simulink model "power_hvdc12pulse"  (Simulink 6.0)
settings: Solver=FixedStepDiscrete  SolverMode=SingleTasking  StartTime=0.0  StopTime=2  FixedStep=Ts  RelTol=1e-3  AbsTol=1e-2
InitFcn:
  | Ts=50e-6;
undefined symbols (not defined in the file or in its folder): CLARK, Current, D1, Delta, DiscIntNeverNeededParam, Gamma, Inverter, lag, lib_mesures, Voltage, Yg
libraries: powerlib x39, powerlib_extras x30, simulink x3
(part 2 of 3)

== system power_hvdc12pulse/Inverter Control and Protection/Inverter Protections ==
  Uabc (pu) : Inport  Port=1  LatchInput=off
  1st-Order T=3.3 ms : powerlib_extras/Discrete  Control Blocks/Discrete 1st-Order Discrete Filter  FilterType=Lowpass  Tc=0.0033  Ts=Ts  Initialize=off  Vac_Init=[0.8 -25 60]  Vdc_Init=-0.4  PlotResponse=off  param1=[1 500 0.1]
  Commutation Failure Prevention Control (CFPREV) : Subsystem  mask(Commutation Failure Prevention Control){STATE=on, T_ss=0.64, ab_level=0.1, ab_gain=25, z_level=0.1, z_gain=25, fn=60, Filter=[2.0, 1.0], Ts=Ts}
      mask prompts: STATE "ON State"; T_ss "Simulation Steady_State Time (s):"; ab_level "ab level (pu):"; ab_gain "ab gain (deg/pu):"; z_level "z level (pu):"; z_gain "z gain (deg/pu):"; fn "Base frequency (Hz):"; Filter "Filter Time const. and Iinitial condition [T(s), Ic (pu)]:"; Ts "Sample Time (s):"
      mask help:
      | The protective function, used in the inverter, mitigates commutation failures due to AC voltage dips. After a fault detection (three-phase or one-phase) an angle value (AMIN_CFPREV) is sent to the converter control in order to be deducted from the maximum delay angle limit (alpha_max). Practicaly, the commutation margin is consequently enlarged reducing therfore the risk of commutation failures.
      |
      |      The CLARK transformation is used for three-phase fault  detection and the zero-sequence voltage evaluation. The detection is based  on instantaneous values, which ensure fast reaction of the control system when AC faults occurs.
      |
      |      Press Help to get the reference with the  detailed description of the function and  parameters.
      |
      | Note: To accelerate the function initialisation, the first parameter (Simulation Steady_State Time) is used. It corresponds to the time when the input voltages reache  the steady-state value.
      mask init:
      | T_periode = 0.6/fn;    % More then half the period
      | filt_tc = Filter(1);
      | filt_ic = Filter(2);
      | 
      | if (STATE)
      | 	str = 'ON';
      | else
      | 	str = 'OFF';
      | end
      mask Help:
      | Ref. "A Novel Method to Mitigate Commutation Failures in HVDC Systems,"
      | Lidong Zhang, Lars Dofnas ABB Utilities Power System Technology,
      | Proceedings PowerCon 2002, Volume: 1 , 13-17 Oct. 2002,  Page(s): 51-56 vol.1.
      mask Display: disp(['\n\n\n State:[',str,']'])
  Informations : Subsystem
      mask Display: disp('?')
  Low AC Voltage Detection (LACVD) : Subsystem  TreatAsAtomicUnit=on  mask(Low AC voltage detection){STATE=on, Ref_1=0.75, dt=fix(0.001/Ts)*Ts}
      mask prompts: STATE "ON State"; Ref_1 "Detection level (pu):"; dt "Sample time (s):"
      mask help:
      | This bloc detects a low AC voltage condition on the commutation busbar and is used in the DC protection scheme. Its purpose is to descriminate between a drop in the AC voltage caused by a fault on the DC line or by a fault on the AC side.
      |
      |      An AC fault detection (Low_ac_voltage output signal) will occur when the AC voltage input (recified three-phase AC voltage) drops below a certain reference value (Detection
      | level).
      |
      |      In order to minimize the simulation time, an enabled susbystem having a sample time of 1 (ms) has been used in accordance with an acceptable precision.
      mask init:
      | if (STATE)
      | 	str = 'ON';
      | else
      | 	str = 'OFF';
      | end
      mask Display: disp(['\n\n\n\nState:[',str,']'])
  T = 1 ms : DiscretePulseGenerator  Period=fix(0.001/Ts)  SampleTime=Ts
  Udio_6p : Subsystem
  Low_AC_Voltage : Outport
  AMIN_CFPREV : Outport  Port=2
  wires:
  T = 1 ms/1 -> Low AC Voltage Detection (LACVD)/Enable
  1st-Order T=3.3 ms/1 -> Low AC Voltage Detection (LACVD)/1(Uac (pu))
  Udio_6p/1(Udio_6p) -> 1st-Order T=3.3 ms/1
  Uabc (pu)/1 -> Commutation Failure Prevention Control (CFPREV)/1(Uabc (pu)), Udio_6p/1(Uabc (pu))
  Low AC Voltage Detection (LACVD)/1(Low_AC_Voltage) -> Low_AC_Voltage/1
  Commutation Failure Prevention Control (CFPREV)/1(AMIN_CFPREV (deg)) -> AMIN_CFPREV/1

== system power_hvdc12pulse/Master Control/Informations ==
  note: For testing purpose,  a step can be activated and added to the reference current at both
      | converters.
  note: Master Control
  note: INTRODUCTION
  note: The rectifier and inverter current reference are generated in the master control. The reference
      | should be equal in both converters to avoid the loss of the margin. The converter starting and stopping is
      | initiated and the current reference can be ramped up or down.  A current step can be added to the
      | current reference for testing purpose.
  note: DESCRIPTION
  note: At start-up, both converters are deblocked and ramped up to the minimum current allowed in steady-state
      | with an adjustable rate  and application time in the "Start/Stop & Ramping Unit" subsystem. After the
      | system stabilisation the current is ramped up to its final value  with an adjustable rate and execution time.
      | Before stopping the converters the current is ramped down to the minimum reference.

== system power_hvdc12pulse/Master Control/Start/Stop ==
  note: Start/Stop sequence
  note: Start/Stop & Ramping
  note: Ramping
  Discrete Bistable : powerlib_extras/Discrete  Control Blocks/Discrete Bistable  Priority=0  ic=0  Ts=50e-6
  Discrete Edge Detector1 : powerlib_extras/Discrete  Control Blocks/Discrete Edge Detector  model=Rising  ic=0  Ts=Ts
  Discrete Edge Detector2 : powerlib_extras/Discrete  Control Blocks/Discrete Edge Detector  model=Rising  ic=0  Ts=Ts
  Logical Operator3 : Logic  AllPortsSameDT=off
  Minimum ref : Constant  Value=Min_ref
  Relational Operator1 : RelationalOperator  Operator=<=
  S1 : Subsystem  mask(RAMPING UNIT){Min_ref=Min_ref, SS_ramp=SS_ramp, F_up=F_up, up_slope=up_slope, T_up=T_up, F_down=F_down, down_slope=down_slope, T_down=T_down}
      mask prompts: Min_ref "Minimum Value (pu):"; SS_ramp "Start-Stop ramp (pu/s):"; F_up "Final Up Value (pu):"; up_slope "Up Slope (pu/s):"; T_up "Ramping Up Time (s):"; F_down "Final Down Value (pu):"; down_slope "Down Slope (pu/s):"; T_down "Ramping Down Time (s):"
      mask init:
      | T_up_final      =  T_up + (F_up - Min_ref)/up_slope;
      | T_down_final =   T_down + (F_down-F_up)/down_slope;
      | T_ramp  = [0, T_up, T_up_final,  T_down,  T_down_final, 9999]';
      | U_ramp = [0, 0, F_up-Min_ref,  F_up-Min_ref,  F_down- Min_ref,  F_down - Min_ref]';
      mask Display: disp('Ramping\n Unit')
  Start : Step  Time=T_start  SampleTime=0
  Stop : Step  Time=T_stop  SampleTime=0
  Unit Delay : UnitDelay  Orientation=left  SampleTime=Ts
  Id_ref_ramp : Outport
  "Stop " : Outport  Port=2
  wires:
  Discrete Edge Detector2/1 -> Discrete Bistable/2
  S1/1(Out1) -> Unit Delay/1, Id_ref_ramp/1
  Discrete Bistable/2 -> "Stop "/1
  Minimum ref/1 -> Relational Operator1/2
  Unit Delay/1 -> Relational Operator1/1
  Start/1 -> Discrete Edge Detector1/1
  Discrete Bistable/1 -> S1/1(Start)  "Start"
  Logical Operator3/1 -> Discrete Edge Detector2/1
  Relational Operator1/1 -> Logical Operator3/1
  Stop/1 -> Logical Operator3/2
  Discrete Edge Detector1/1 -> Discrete Bistable/1

== system power_hvdc12pulse/Rectifier/Rectifier ==
  Py : Inport  Port=1  LatchInput=off
  Pd : Inport  Port=2  LatchInput=off
  Bridge D : powerlib/Power Electronics/Universal Bridge  Arms=3  SnubberResistance=2000  SnubberCapacitance=0.1e-6  Device=Thyristors  Ron=1e-3  Lon=0  ForwardVoltages="[  0.8  0.8  ]"  ForwardVoltage=0  GTOparameters=[ 10e-6 , 20e-6 ]  IGBTparameters=[ 1e-6 , 2e-6 ]  Measurements=None
  Bridge Y : powerlib/Power Electronics/Universal Bridge  Arms=3  SnubberResistance=2000  SnubberCapacitance=0.1e-6  Device=Thyristors  Ron=1e-3  Lon=0  ForwardVoltages="[  0.8  0.8  ]"  ForwardVoltage=0  GTOparameters=[ 10e-6 , 20e-6 ]  IGBTparameters=[ 1e-6 , 2e-6 ]  Measurements=All voltages and currents
  Ay : PMIOPort  Port=1  Side=Left
  By : PMIOPort  Port=2  Side=Left
  Cy : PMIOPort  Port=3  Side=Left
  Ad : PMIOPort  Port=4  Side=Left
  Bd : PMIOPort  Port=5  Side=Left
  Cd : PMIOPort  Port=6  Side=Left
  pos : PMIOPort  Orientation=left  Port=7  Side=Right
  neg : PMIOPort  Orientation=left  Port=8  Side=Right
  wires:
  Pd/1 -> Bridge D/1
  Py/1 -> Bridge Y/1
  connections:
  Bridge D/RConn2 -- neg/RConn1
  Cd/RConn1 -- Bridge D/LConn3
  Bd/RConn1 -- Bridge D/LConn2
  Ad/RConn1 -- Bridge D/LConn1
  Cy/RConn1 -- Bridge Y/LConn3
  By/RConn1 -- Bridge Y/LConn2
  Bridge Y/RConn1 -- pos/RConn1
  Ay/RConn1 -- Bridge Y/LConn1
  Bridge D/RConn1 -- Bridge Y/RConn2

== system power_hvdc12pulse/Rectifier Control and Protection/12-pulse Firing Control1 ==
  alpha_ord (deg) : Inport  Port=1  LatchInput=off
  Vabc (pu) : Inport  Port=2  LatchInput=off
  Block : Inport  Port=3  LatchInput=off
  Discrete Synchronized 12-Pulse Generator : Subsystem  AncestorBlock=|  mask(Discrete synchronized 12-pulse generator){pwidth=Pw, Double_Pulse=off, Ts=dt}
      | powerlib_extras/Discrete 
      | Control Blocks/Discrete Synchronized
      | 12-Pulse Generator
      mask prompts: pwidth "Pulse width (degrees) :"; Double_Pulse "Double pulsing"; Ts "Sample time:"
      mask help:
      | Use his block  to fire the 12 thyristors of a 12-pulse converter.
      | Outputs 1 and 2 are two vectors of 6 pulses (0-1) to be sent to the two 6-pulse half bridges connected respectively to the Wye(Y) and Delta (D) connected windings of the YYD converter transformer. Pulses are individually synchronized on the 6 commutation voltages and generated alpha degrees after the increasing zero-crossings of the commutation voltages. The D pulses are lagging the Y pulses by  60 degrees.
      |
      | Input 1 is  the alpha firing signal (degrees).
      | Inputs 2, 3 and 4 are the three phase-ground synchronization voltages  measured at the  primary side of the converter transformer.
      | Input 5: Frequency of the synchronization voltages (use a constant or the Freq PLL output)
      | Input 6 allows  blocking of the pulses when the applied signal is non zero.
      |
      | When the 'Douple pulsing' option is checked, two pulses are sent to each thyristor: a 1st pulse when the aplha angle is reached, then a 2nd pulse 60 degrees later, when the next thyristor is fired.
      mask Display: plot(0,0,100,100,[80 62 62 47 47 30],[40 40 60 60 40 40]-5)
  PLL : Subsystem
  PulsesY : Outport
  PulsesD : Outport  Port=2
  Freq : Outport  Port=3
  wires:
  Discrete Synchronized 12-Pulse Generator/1(PY) -> PulsesY/1
  Discrete Synchronized 12-Pulse Generator/2(PD) -> PulsesD/1
  Vabc (pu)/1 -> PLL/1(Vabc(pu))
  PLL/1(Va) -> Discrete Synchronized 12-Pulse Generator/2(A)
  PLL/2(Vb) -> Discrete Synchronized 12-Pulse Generator/3(B)
  PLL/3(Vc) -> Discrete Synchronized 12-Pulse Generator/4(C)
  PLL/4(Freq) -> Discrete Synchronized 12-Pulse Generator/5(Freq), Freq/1
  alpha_ord (deg)/1 -> Discrete Synchronized 12-Pulse Generator/1(alpha_deg)
  Block/1 -> Discrete Synchronized 12-Pulse Generator/6(Block)

== system power_hvdc12pulse/Rectifier Control and Protection/Rectifier Protections ==
  note: DC Protections (in Rectifier)
  Uabc (pu) : Inport  Port=1  LatchInput=off
  VdL (pu) : Inport  Port=2  LatchInput=off
  Deblocked : Inport  Port=3  LatchInput=off
  Low_ac_volt_oth : Inport  Port=4  LatchInput=off
  1st-Order T=3.3 ms : powerlib_extras/Discrete  Control Blocks/Discrete 1st-Order Discrete Filter  FilterType=Lowpass  Tc=0.0033  Ts=Ts  Initialize=off  Vac_Init=[0.8 -25 60]  Vdc_Init=-0.4  PlotResponse=off  param1=[1 500 0.1]
  DC Fault Protection (DCPROT) : Subsystem  mask(DC fault protection (in Rectifier)){STATE=on, Ref1=0.5, T1=0.070, T2=0.05, polarity=Positive, dt=fix(0.002/Ts)*Ts}
      mask prompts: STATE "ON State"; Ref1 "Detection level (pu):"; T1 "Detection delay (s):"; T2 "Forced alpha duration (s):"; polarity "Voltage polarity:"; dt "Sample time (s):"
      mask help:
      | The protection is active in the rectifier. It will detect a fault on the DC side and will force the delay angle into the inverter region in order to extinguish the fault current.
      |      The fault detection on the DC line is based on the drop in the line to ground voltage.
      |      The normal voltage polarity (+ or -) of the line is a parameter as well as the reference level (Detection level) of the fault detection.
      |      A delay time (Detection delay) is used in the detection to descriminate between a line fault and other disturbances resulting in a low DC voltage.
      |      A delay time (200 ms) is allowed, after the DC system start-up, before activating the detection logic to make sure that the normal operating DC voltage is established.
      |      Also, an external signal (Lock) generated by another protective function (e.g. Low AC voltage detection) will lock the detection for a minimum amount of time (set by an Off Delay bloc) in order to descriminate between any fault causing a low DC voltage.
      |      A detection will triger a Forced alpha during an ajustable interval (Forced alpha duration) sufficient to allow for deionization of the fault path prior to re-application of voltage.
      |
      |      In order to minimize the simulation time, an enabled susbystem having a sample time of  2 (ms) has been used in accordance with an acceptable precision.
      mask init:
      | if (polarity == 1)
      | 	sign = 1;
      | else
      | 	sign = -1;
      | end
      | 
      | if (STATE)
      | 	str = 'ON';
      | else
      | 	str = 'OFF';
      | end
      mask StyleString: checkbox,edit,edit,edit,popup(Positive|Negative),edit
      mask Display: disp(['\n\n\n\nState:[',str,']'])
  Informations : Subsystem
      mask Display: disp('?')
  Logical Operator6 : Logic  Operator=OR
  Low AC Voltage Detection (LACVD) : Subsystem  TreatAsAtomicUnit=on  mask(Low AC voltage detection){STATE=on, Ref_1=0.70, dt=fix(0.001/Ts)*Ts}
      mask prompts: STATE "ON State"; Ref_1 "Detection level (pu):"; dt "Sample time (s):"
      mask help:
      | This bloc detects a low AC voltage condition on the commutation busbar and is used in the DC protection scheme. Its purpose is to descriminate between a drop in the AC voltage caused by a fault on the DC line or by a fault on the AC side.
      |
      |      An AC fault detection (Low_ac_voltage output signal) will occur when the AC voltage input (recified three-phase AC voltage) drops below a certain reference value (Detection level).
      |
      |      In order to minimize the simulation time, an enabled susbystem having a sample time of 1 (ms) has been used in accordance with an acceptable precision.
      mask init:
      | if (STATE)
      | 	str = 'ON';
      | else
      | 	str = 'OFF';
      | end
      mask Display: disp(['\n\n\n\nState:[',str,']'])
  T = 1 ms : DiscretePulseGenerator  Period=fix(0.001/Ts)  SampleTime=Ts
  T = 2 ms : DiscretePulseGenerator  Period=fix(0.002/Ts)  SampleTime=Ts
  Udio_6p : Subsystem
  Forced_alpha : Outport
  Low_ac_voltage : Outport  Port=2
  wires:
  T = 1 ms/1 -> Low AC Voltage Detection (LACVD)/Enable
  1st-Order T=3.3 ms/1 -> Low AC Voltage Detection (LACVD)/1(Uac (pu))
  Udio_6p/1(Udio_6p) -> 1st-Order T=3.3 ms/1
  Uabc (pu)/1 -> Udio_6p/1(Uabc (pu))
  Low AC Voltage Detection (LACVD)/1(Low_AC_Voltage) -> Logical Operator6/1, Low_ac_voltage/1
  T = 2 ms/1 -> DC Fault Protection (DCPROT)/Enable
  DC Fault Protection (DCPROT)/1(Forced_alpha) -> Forced_alpha/1
  Low_ac_volt_oth/1 -> Logical Operator6/2
  Logical Operator6/1 -> DC Fault Protection (DCPROT)/3(Lock)
  VdL (pu)/1 -> DC Fault Protection (DCPROT)/1(VdL (pu))
  Deblocked/1 -> DC Fault Protection (DCPROT)/2(Deblocked)

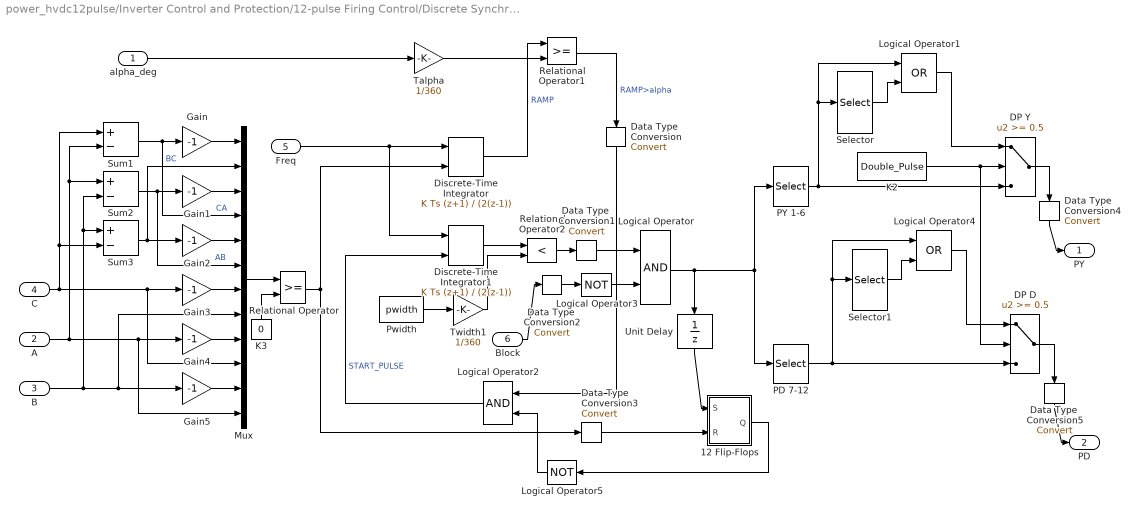
== system power_hvdc12pulse/Inverter Control and Protection/12-pulse Firing Control/Discrete Synchronized 12-Pulse Generator ==
  alpha_deg : Inport  Port=1  LatchInput=off
  A : Inport  Port=2  LatchInput=off
  B : Inport  Port=3  LatchInput=off
  C : Inport  Port=4  LatchInput=off
  Freq : Inport  Port=5  LatchInput=off
  Block : Inport  Port=6  LatchInput=off
  12 Flip-Flops : Subsystem
  DP D : Switch  Threshold=0.5  InputSameDT=on
  DP Y : Switch  Threshold=0.5  InputSameDT=on
  Data Type  Conversion : DataTypeConversion  Orientation=down  OutDataTypeMode=boolean  SaturateOnIntegerOverflow=on  RndMeth=Zero
  Data Type  Conversion1 : DataTypeConversion  OutDataTypeMode=boolean  SaturateOnIntegerOverflow=on  RndMeth=Zero
  Data Type  Conversion2 : DataTypeConversion  OutDataTypeMode=boolean  SaturateOnIntegerOverflow=on  RndMeth=Zero
  Data Type  Conversion3 : DataTypeConversion  OutDataTypeMode=boolean  SaturateOnIntegerOverflow=on  RndMeth=Zero
  Data Type  Conversion4 : DataTypeConversion  Orientation=down  OutDataTypeMode=double  SaturateOnIntegerOverflow=on  RndMeth=Zero
  Data Type  Conversion5 : DataTypeConversion  Orientation=down  OutDataTypeMode=double  SaturateOnIntegerOverflow=on  RndMeth=Zero
  Discrete-Time Integrator : DiscreteIntegrator  IntegratorMethod=Integration: Trapezoidal  ExternalReset=rising  SampleTime=Ts  ICPrevOutput=DiscIntNeverNeededParam  ICPrevScaledInput=DiscIntNeverNeededParam
  Discrete-Time Integrator1 : DiscreteIntegrator  IntegratorMethod=Integration: Trapezoidal  ExternalReset=rising  SampleTime=Ts  ICPrevOutput=DiscIntNeverNeededParam  ICPrevScaledInput=DiscIntNeverNeededParam
  Gain{,1..5} (6 alike) : Gain  Gain=-1  SaturateOnIntegerOverflow=on
  K2 : Constant  Value=Double_Pulse
  K3 : Constant  Orientation=up  Value=0
  Logical Operator : Logic
  Logical Operator1 : Logic  Operator=OR
  Logical Operator2 : Logic  Orientation=left
  Logical Operator3 : Logic  Operator=NOT  Inputs=1
  Logical Operator4 : Logic  Operator=OR
  Logical Operator5 : Logic  Orientation=left  Operator=NOT  Inputs=1
  Mux : Mux  Inputs=12
  PD 7-12 : Selector  Elements=7:12  InputPortWidth=12
  PY 1-6 : Selector  Elements=1:6  InputPortWidth=12
  Pwidth : Constant  Value=pwidth
  Relational Operator : RelationalOperator  InputSameDT=on
  Relational Operator1 : RelationalOperator  InputSameDT=on
  Relational Operator2 : RelationalOperator  Operator=<  InputSameDT=on
  Selector : Selector  Elements=[2 3 4 5 6 1 ]  InputPortWidth=6
  Selector1 : Selector  Elements=[2 3 4 5 6 1 ]  InputPortWidth=6
  Sum1 : Sum  Inputs=+-  SaturateOnIntegerOverflow=on  InputSameDT=on
  Sum2 : Sum  Inputs=+-  SaturateOnIntegerOverflow=on  InputSameDT=on
  Sum3 : Sum  Inputs=+-  SaturateOnIntegerOverflow=on  InputSameDT=on
  Talpha : Gain  Gain=1/360  SaturateOnIntegerOverflow=on
  Twidth1 : Gain  Gain=1/360  SaturateOnIntegerOverflow=on
  Unit Delay : UnitDelay  Orientation=down  SampleTime=Ts
  PY : Outport  InitialOutput=0
  PD : Outport  Port=2  InitialOutput=0
  wires:
  Freq/1 -> Discrete-Time Integrator1/1, Discrete-Time Integrator/1
  K3/1 -> Relational Operator/2
  Mux/1 -> Relational Operator/1
  Gain2/1 -> Mux/5
  Gain1/1 -> Mux/3
  Gain/1 -> Mux/1
  alpha_deg/1 -> Talpha/1
  Sum1/1 -> Gain/1, Mux/4  "CA"
  Sum2/1 -> Gain1/1, Mux/6  "AB"
  Sum3/1 -> Gain2/1, Mux/2  "BC"
  Gain3/1 -> Mux/7
  Gain4/1 -> Mux/9
  Gain5/1 -> Mux/11
  C/1 -> Gain3/1, Mux/10, Sum1/1, Sum3/2
  A/1 -> Gain4/1, Mux/12, Sum2/1, Sum1/2
  B/1 -> Gain5/1, Mux/8, Sum3/1, Sum2/2
  Discrete-Time Integrator/1 -> Relational Operator1/1  "RAMP"
  Talpha/1 -> Relational Operator1/2
  Discrete-Time Integrator1/1 -> Relational Operator2/1
  Twidth1/1 -> Relational Operator2/2
  Logical Operator2/1 -> Discrete-Time Integrator1/2  "START_PULSE"
  Logical Operator5/1 -> Logical Operator2/2
  Relational Operator/1 -> Discrete-Time Integrator/2, Data Type  Conversion3/1
  Pwidth/1 -> Twidth1/1
  Logical Operator3/1 -> Logical Operator/2
  12 Flip-Flops/1(Q) -> Logical Operator5/1
  Logical Operator/1 -> Unit Delay/1, PY 1-6/1, PD 7-12/1
  Logical Operator1/1 -> DP Y/1
  Selector/1 -> Logical Operator1/2
  PY 1-6/1 -> DP Y/3, Selector/1, Logical Operator1/1
  Logical Operator4/1 -> DP D/1
  Selector1/1 -> Logical Operator4/2
  PD 7-12/1 -> Logical Operator4/1, Selector1/1, DP D/3
  K2/1 -> DP Y/2, DP D/2
  Unit Delay/1 -> 12 Flip-Flops/1(S)
  Relational Operator1/1 -> Data Type  Conversion/1  "RAMP>alpha"
  Data Type  Conversion/1 -> Logical Operator2/1
  Relational Operator2/1 -> Data Type  Conversion1/1
  Data Type  Conversion1/1 -> Logical Operator/1
  Block/1 -> Data Type  Conversion2/1
  Data Type  Conversion2/1 -> Logical Operator3/1
  Data Type  Conversion3/1 -> 12 Flip-Flops/2(R)
  DP Y/1 -> Data Type  Conversion4/1
  Data Type  Conversion4/1 -> PY/1
  DP D/1 -> Data Type  Conversion5/1
  Data Type  Conversion5/1 -> PD/1

== system power_hvdc12pulse/Inverter Control and Protection/12-pulse Firing Control/PLL ==
  Vabc(pu) : Inport  Port=1  LatchInput=off
  Constant : Constant  Value=2*pi/3
  Discrete 3-phase PLL : powerlib_extras/Discrete  Control Blocks/Discrete 3-phase PLL  Fmin=0.75 * PLL_f0  Par_Init="[PLL_ph  PLL_f0]"  ParK="[PLL_Kp  PLL_Ki]"  Ts=dt
  Sum : Sum  Inputs=|+-  SaturateOnIntegerOverflow=on
  Sum1 : Sum  Inputs=|++  SaturateOnIntegerOverflow=on
  Terminator : Terminator
  Trigonometric Function : Trigonometry
  Trigonometric Function1 : Trigonometry
  Trigonometric Function2 : Trigonometry
  Va : Outport
  Vb : Outport  Port=2
  Vc : Outport  Port=3
  Freq : Outport  Port=4
  wires:
  Discrete 3-phase PLL/1 -> Freq/1
  Vabc(pu)/1 -> Discrete 3-phase PLL/1
  Discrete 3-phase PLL/2 -> Trigonometric Function/1, Sum/1, Sum1/1
  Sum/1 -> Trigonometric Function1/1
  Constant/1 -> Sum1/2, Sum/2
  Sum1/1 -> Trigonometric Function2/1
  Trigonometric Function/1 -> Va/1
  Trigonometric Function1/1 -> Vb/1
  Trigonometric Function2/1 -> Vc/1
  Discrete 3-phase PLL/3 -> Terminator/1

== system power_hvdc12pulse/Inverter Control and Protection/Inverter Protections/Commutation Failure Prevention Control (CFPREV) ==
  note: Commutation failure Prevention Control Module (CFPREV)
  Uabc (pu) : Inport  Port=1  LatchInput=off
  C : Constant  Value=STATE
  Enabled Subsystem : Subsystem  TreatAsAtomicUnit=on
  AMIN_CFPREV (deg) : Outport
  wires:
  C/1 -> Enabled Subsystem/Enable
  Uabc (pu)/1 -> Enabled Subsystem/1(Uabc (pu))
  Enabled Subsystem/1(AMIN_CFPREV (deg)) -> AMIN_CFPREV (deg)/1

== system power_hvdc12pulse/Inverter Control and Protection/Inverter Protections/Informations ==
  note: The CFPREV  mitigates commutation failures due to AC voltage dips. After a fault detection (three-phase or
      | one-phase) an angle value (AMIN_CFPREV) is sent to the converter control in order to be deducted from the
      | maximum delay angle limit (alpha_max). In practice, the commutation margin is consequently enlarged
      | reducing therefore the risk of commutation failures (note 1).
  note: The Commutation failure prevention control (CFPREV) and the Low AC voltage detection (LACVD)
      | constitutes the protective functions at the rinverter.
  note: The LACVD detects a low AC voltage condition on the inverter commutation bus and sends a signal
      | (Lock) to the DCPROT (in the rectifier) in order to prevent the detection of a DC fault when the drop in
      | the DC voltage is due to a fault on the AC side. The LACVD at the irectifier sends also a signal to
      | lock the DCPROT for the same reason.
  note: DESCRIPTION
  note: DC Protections - Inverter
  note: NOTE 1: Result of a failure of the incoming valve to take over the direct current before the commutating voltage reverses its polarity.

== system power_hvdc12pulse/Inverter Control and Protection/Inverter Protections/Low AC Voltage Detection (LACVD) ==
  note: Low AC Voltage Detection
  Uac (pu) : Inport  Port=1  LatchInput=off
  cycle = 1 (ms) : EnablePort  ShowOutputPort=on
  C : Constant  Value=STATE
  Enabled Subsystem : Subsystem  TreatAsAtomicUnit=on
  Logical Operator : Logic  AllPortsSameDT=off
  Low_AC_Voltage : Outport
  wires:
  Uac (pu)/1 -> Enabled Subsystem/1(Uac (pu))
  Enabled Subsystem/1(Low_AC_Voltage) -> Low_AC_Voltage/1
  cycle = 1 (ms)/1 -> Logical Operator/1
  Logical Operator/1 -> Enabled Subsystem/Enable
  C/1 -> Logical Operator/2

== system power_hvdc12pulse/Inverter Control and Protection/Inverter Protections/Udio_6p ==
  note: Silvano Casoria
      | Power System Laboratory, IREQ
      | Hydro-Quebec
  note: Three-phase full-wave rectification
  Uabc (pu) : Inport  Port=1  LatchInput=off
  MinMax : MinMax  Function=max  SaturateOnIntegerOverflow=on  InputSameDT=on
  MinMax1 : MinMax  SaturateOnIntegerOverflow=on  InputSameDT=on
  Sum : Sum  Inputs=+-  SaturateOnIntegerOverflow=on  InputSameDT=on
  conversion pu ac->dc : Gain  Gain=pi/(3*sqrt(3))  SaturateOnIntegerOverflow=on
  Udio_6p : Outport
  wires:
  MinMax1/1 -> Sum/2
  MinMax/1 -> Sum/1
  Uabc (pu)/1 -> MinMax/1, MinMax1/1
  Sum/1 -> conversion pu ac->dc/1
  conversion pu ac->dc/1 -> Udio_6p/1

== system power_hvdc12pulse/Master Control/Start/Stop/S1 ==
  Start : Inport  Port=1  LatchInput=off
  Down : Constant  Value=0
  Ramp : FromWorkspace  VariableName="[T_ramp,  U_ramp]"  SampleTime=Ts
  Start-Stop Ramp : RateLimiter  RisingSlewLimit=SS_ramp  FallingSlewLimit=-SS_ramp
  Sum : Sum  SaturateOnIntegerOverflow=on  InputSameDT=on
  Switch : Switch  Threshold=0.5  SaturateOnIntegerOverflow=on
  UP : Constant  Value=Min_ref
  Out1 : Outport  InitialOutput=0
  wires:
  Sum/1 -> Out1/1
  Ramp/1 -> Sum/1
  Start/1 -> Switch/2
  Switch/1 -> Start-Stop Ramp/1
  Down/1 -> Switch/3
  UP/1 -> Switch/1
  Start-Stop Ramp/1 -> Sum/2

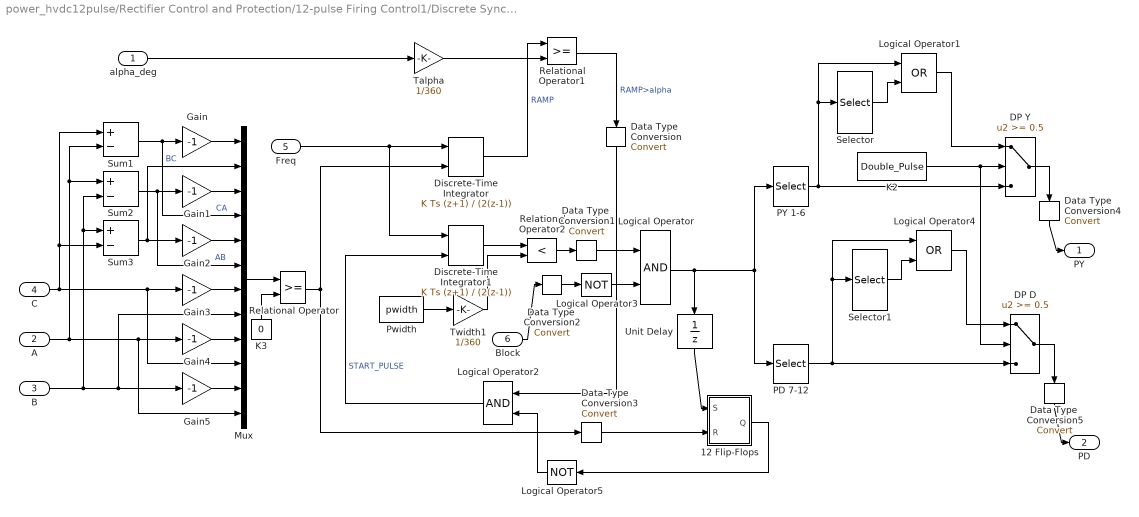
== system power_hvdc12pulse/Rectifier Control and Protection/12-pulse Firing Control1/Discrete Synchronized 12-Pulse Generator ==
  alpha_deg : Inport  Port=1  LatchInput=off
  A : Inport  Port=2  LatchInput=off
  B : Inport  Port=3  LatchInput=off
  C : Inport  Port=4  LatchInput=off
  Freq : Inport  Port=5  LatchInput=off
  Block : Inport  Port=6  LatchInput=off
  12 Flip-Flops : Subsystem
  DP D : Switch  Threshold=0.5  InputSameDT=on
  DP Y : Switch  Threshold=0.5  InputSameDT=on
  Data Type  Conversion : DataTypeConversion  Orientation=down  OutDataTypeMode=boolean  SaturateOnIntegerOverflow=on  RndMeth=Zero
  Data Type  Conversion1 : DataTypeConversion  OutDataTypeMode=boolean  SaturateOnIntegerOverflow=on  RndMeth=Zero
  Data Type  Conversion2 : DataTypeConversion  OutDataTypeMode=boolean  SaturateOnIntegerOverflow=on  RndMeth=Zero
  Data Type  Conversion3 : DataTypeConversion  OutDataTypeMode=boolean  SaturateOnIntegerOverflow=on  RndMeth=Zero
  Data Type  Conversion4 : DataTypeConversion  Orientation=down  OutDataTypeMode=double  SaturateOnIntegerOverflow=on  RndMeth=Zero
  Data Type  Conversion5 : DataTypeConversion  Orientation=down  OutDataTypeMode=double  SaturateOnIntegerOverflow=on  RndMeth=Zero
  Discrete-Time Integrator : DiscreteIntegrator  IntegratorMethod=Integration: Trapezoidal  ExternalReset=rising  SampleTime=Ts  ICPrevOutput=DiscIntNeverNeededParam  ICPrevScaledInput=DiscIntNeverNeededParam
  Discrete-Time Integrator1 : DiscreteIntegrator  IntegratorMethod=Integration: Trapezoidal  ExternalReset=rising  SampleTime=Ts  ICPrevOutput=DiscIntNeverNeededParam  ICPrevScaledInput=DiscIntNeverNeededParam
  Gain{,1..5} (6 alike) : Gain  Gain=-1  SaturateOnIntegerOverflow=on
  K2 : Constant  Value=Double_Pulse
  K3 : Constant  Orientation=up  Value=0
  Logical Operator : Logic
  Logical Operator1 : Logic  Operator=OR
  Logical Operator2 : Logic  Orientation=left
  Logical Operator3 : Logic  Operator=NOT  Inputs=1
  Logical Operator4 : Logic  Operator=OR
  Logical Operator5 : Logic  Orientation=left  Operator=NOT  Inputs=1
  Mux : Mux  Inputs=12
  PD 7-12 : Selector  Elements=7:12  InputPortWidth=12
  PY 1-6 : Selector  Elements=1:6  InputPortWidth=12
  Pwidth : Constant  Value=pwidth
  Relational Operator : RelationalOperator  InputSameDT=on
  Relational Operator1 : RelationalOperator  InputSameDT=on
  Relational Operator2 : RelationalOperator  Operator=<  InputSameDT=on
  Selector : Selector  Elements=[2 3 4 5 6 1 ]  InputPortWidth=6
  Selector1 : Selector  Elements=[2 3 4 5 6 1 ]  InputPortWidth=6
  Sum1 : Sum  Inputs=+-  SaturateOnIntegerOverflow=on  InputSameDT=on
  Sum2 : Sum  Inputs=+-  SaturateOnIntegerOverflow=on  InputSameDT=on
  Sum3 : Sum  Inputs=+-  SaturateOnIntegerOverflow=on  InputSameDT=on
  Talpha : Gain  Gain=1/360  SaturateOnIntegerOverflow=on
  Twidth1 : Gain  Gain=1/360  SaturateOnIntegerOverflow=on
  Unit Delay : UnitDelay  Orientation=down  SampleTime=Ts
  PY : Outport  InitialOutput=0
  PD : Outport  Port=2  InitialOutput=0
  wires:
  Freq/1 -> Discrete-Time Integrator1/1, Discrete-Time Integrator/1
  K3/1 -> Relational Operator/2
  Mux/1 -> Relational Operator/1
  Gain2/1 -> Mux/5
  Gain1/1 -> Mux/3
  Gain/1 -> Mux/1
  alpha_deg/1 -> Talpha/1
  Sum1/1 -> Gain/1, Mux/4  "CA"
  Sum2/1 -> Gain1/1, Mux/6  "AB"
  Sum3/1 -> Gain2/1, Mux/2  "BC"
  Gain3/1 -> Mux/7
  Gain4/1 -> Mux/9
  Gain5/1 -> Mux/11
  C/1 -> Gain3/1, Mux/10, Sum1/1, Sum3/2
  A/1 -> Gain4/1, Mux/12, Sum2/1, Sum1/2
  B/1 -> Gain5/1, Mux/8, Sum3/1, Sum2/2
  Discrete-Time Integrator/1 -> Relational Operator1/1  "RAMP"
  Talpha/1 -> Relational Operator1/2
  Discrete-Time Integrator1/1 -> Relational Operator2/1
  Twidth1/1 -> Relational Operator2/2
  Logical Operator2/1 -> Discrete-Time Integrator1/2  "START_PULSE"
  Logical Operator5/1 -> Logical Operator2/2
  Relational Operator/1 -> Discrete-Time Integrator/2, Data Type  Conversion3/1
  Pwidth/1 -> Twidth1/1
  Logical Operator3/1 -> Logical Operator/2
  12 Flip-Flops/1(Q) -> Logical Operator5/1
  Logical Operator/1 -> Unit Delay/1, PY 1-6/1, PD 7-12/1
  Logical Operator1/1 -> DP Y/1
  Selector/1 -> Logical Operator1/2
  PY 1-6/1 -> DP Y/3, Selector/1, Logical Operator1/1
  Logical Operator4/1 -> DP D/1
  Selector1/1 -> Logical Operator4/2
  PD 7-12/1 -> Logical Operator4/1, Selector1/1, DP D/3
  K2/1 -> DP Y/2, DP D/2
  Unit Delay/1 -> 12 Flip-Flops/1(S)
  Relational Operator1/1 -> Data Type  Conversion/1  "RAMP>alpha"
  Data Type  Conversion/1 -> Logical Operator2/1
  Relational Operator2/1 -> Data Type  Conversion1/1
  Data Type  Conversion1/1 -> Logical Operator/1
  Block/1 -> Data Type  Conversion2/1
  Data Type  Conversion2/1 -> Logical Operator3/1
  Data Type  Conversion3/1 -> 12 Flip-Flops/2(R)
  DP Y/1 -> Data Type  Conversion4/1
  Data Type  Conversion4/1 -> PY/1
  DP D/1 -> Data Type  Conversion5/1
  Data Type  Conversion5/1 -> PD/1

== system power_hvdc12pulse/Rectifier Control and Protection/12-pulse Firing Control1/PLL ==
  Vabc(pu) : Inport  Port=1  LatchInput=off
  Constant : Constant  Value=2*pi/3
  Discrete 3-phase PLL : powerlib_extras/Discrete  Control Blocks/Discrete 3-phase PLL  Fmin=0.75 * PLL_f0  Par_Init="[PLL_ph  PLL_f0]"  ParK="[PLL_Kp  PLL_Ki]"  Ts=dt
  Sum : Sum  Inputs=|+-  SaturateOnIntegerOverflow=on
  Sum1 : Sum  Inputs=|++  SaturateOnIntegerOverflow=on
  Terminator : Terminator
  Trigonometric Function : Trigonometry
  Trigonometric Function1 : Trigonometry
  Trigonometric Function2 : Trigonometry
  Va : Outport
  Vb : Outport  Port=2
  Vc : Outport  Port=3
  Freq : Outport  Port=4
  wires:
  Discrete 3-phase PLL/1 -> Freq/1
  Vabc(pu)/1 -> Discrete 3-phase PLL/1
  Discrete 3-phase PLL/2 -> Trigonometric Function/1, Sum/1, Sum1/1
  Sum/1 -> Trigonometric Function1/1
  Constant/1 -> Sum1/2, Sum/2
  Sum1/1 -> Trigonometric Function2/1
  Trigonometric Function/1 -> Va/1
  Trigonometric Function1/1 -> Vb/1
  Trigonometric Function2/1 -> Vc/1
  Discrete 3-phase PLL/3 -> Terminator/1

== system power_hvdc12pulse/Rectifier Control and Protection/Rectifier Protections/DC Fault Protection (DCPROT) ==
  note: DC Fault Protection (only in Rectifier)
  VdL (pu) : Inport  Port=1  LatchInput=off
  Deblocked : Inport  Port=2  DataType=boolean  LatchInput=off
  Lock : Inport  Port=3  LatchInput=off
  cycle = 2 (ms) : EnablePort  ShowOutputPort=on
  C : Constant  Value=STATE
  Enabled Subsystem : Subsystem  TreatAsAtomicUnit=on
  Logical Operator : Logic  AllPortsSameDT=off
  Forced_alpha : Outport
  wires:
  cycle = 2 (ms)/1 -> Logical Operator/1
  C/1 -> Logical Operator/2
  Logical Operator/1 -> Enabled Subsystem/Enable
  VdL (pu)/1 -> Enabled Subsystem/1(VdL (pu))
  Lock/1 -> Enabled Subsystem/3(Lock)
  Deblocked/1 -> Enabled Subsystem/2(Deblocked)
  Enabled Subsystem/1(Forced_alpha) -> Forced_alpha/1

== system power_hvdc12pulse/Rectifier Control and Protection/Rectifier Protections/Informations ==
  note: The  DCPROT detects a fault on the DC line and tries to extinguish the fault current by ordering a Forced
      | alpha operation for a fixed duration.
  note: The LACVD detects a low AC voltage condition on the rectifier commutation bus and sends a signal
      | (Lock) to the DCPROT in order to prevent the detection of a DC fault when the drop in the DC voltage is
      | due to a fault on the AC side. The LACVD at the inverter sends also a signal to lock the DCPROT for the
      | same reason.
  note: DC Protections - Rectifier
  note: Silvano Casoria (Hydro-Quebec)
  note: DESCRIPTION
  note: The DC fault protection (DCPROT) and the Low AC voltage detection (LACVD) constitutes the
      | protectives functions at the rectifier. The DC fault protection detects a fault on the DC line and tries to
      | extinguish the fault current by ordering a Forced alpha operation during a fixed duration.

== system power_hvdc12pulse/Rectifier Control and Protection/Rectifier Protections/Low AC Voltage Detection (LACVD) ==
  note: Low AC Voltage Detection
  Uac (pu) : Inport  Port=1  LatchInput=off
  cycle = 1 (ms) : EnablePort  ShowOutputPort=on
  C : Constant  Value=STATE
  Enabled Subsystem : Subsystem  TreatAsAtomicUnit=on
  Logical Operator : Logic  AllPortsSameDT=off
  Low_AC_Voltage : Outport
  wires:
  Uac (pu)/1 -> Enabled Subsystem/1(Uac (pu))
  Enabled Subsystem/1(Low_AC_Voltage) -> Low_AC_Voltage/1
  cycle = 1 (ms)/1 -> Logical Operator/1
  Logical Operator/1 -> Enabled Subsystem/Enable
  C/1 -> Logical Operator/2

== system power_hvdc12pulse/Rectifier Control and Protection/Rectifier Protections/Udio_6p ==
  note: Three-phase full-wave rectification
  note: Silvano Casoria
      | Power System Laboratory, IREQ
      | Hydro-Quebec
  Uabc (pu) : Inport  Port=1  LatchInput=off
  MinMax : MinMax  Function=max  SaturateOnIntegerOverflow=on  InputSameDT=on
  MinMax1 : MinMax  SaturateOnIntegerOverflow=on  InputSameDT=on
  Sum : Sum  Inputs=+-  SaturateOnIntegerOverflow=on  InputSameDT=on
  conversion pu ac->dc : Gain  Gain=pi/(3*sqrt(3))  SaturateOnIntegerOverflow=on
  Udio_6p : Outport
  wires:
  conversion pu ac->dc/1 -> Udio_6p/1
  Sum/1 -> conversion pu ac->dc/1
  Uabc (pu)/1 -> MinMax1/1, MinMax/1
  MinMax/1 -> Sum/1
  MinMax1/1 -> Sum/2

== system power_hvdc12pulse/Inverter Control and Protection/12-pulse Firing Control/Discrete Synchronized 12-Pulse Generator/12 Flip-Flops ==
  S : Inport  Port=1  LatchInput=off
  R : Inport  Port=2  LatchInput=off
  6 Flip-Flop : Subsystem
  6 Flip-Flop1 : Subsystem
  Demux : Demux  Outputs=2
  Demux1 : Demux  Outputs=2
  Mux : Mux  Inputs=2
  Q : Outport
  wires:
  S/1 -> Demux/1
  Demux/1 -> 6 Flip-Flop/1(S)
  Demux/2 -> 6 Flip-Flop1/1(S)
  R/1 -> Demux1/1
  Demux1/2 -> 6 Flip-Flop1/2(R)
  Demux1/1 -> 6 Flip-Flop/2(R)
  6 Flip-Flop/1(Q) -> Mux/1
  Mux/1 -> Q/1
  6 Flip-Flop1/1(Q) -> Mux/2

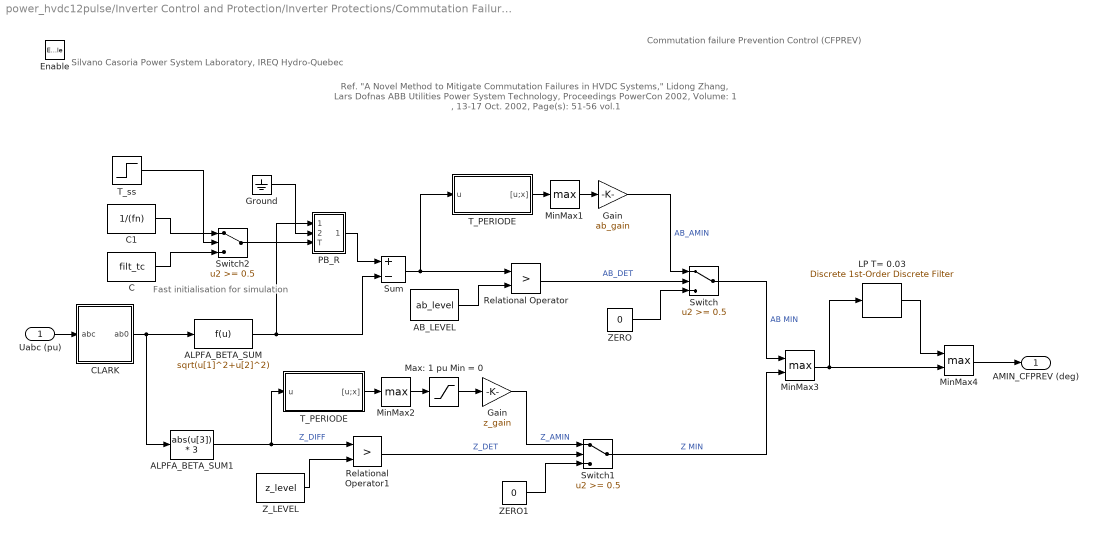
== system power_hvdc12pulse/Inverter Control and Protection/Inverter Protections/Commutation Failure Prevention Control (CFPREV)/Enabled Subsystem ==
  note: Ref. "A Novel Method to Mitigate Commutation Failures in HVDC Systems,"
      | Lidong Zhang, Lars Dofnas ABB Utilities Power System Technology,
      | Proceedings PowerCon 2002, Volume: 1 , 13-17 Oct. 2002,  Page(s): 51-56 vol.1
  note: Silvano Casoria
      | Power System Laboratory, IREQ
      | Hydro-Quebec
  note: Commutation failure Prevention Control (CFPREV)
  note: Fast initialisation
      | for simulation
  Uabc (pu) : Inport  Port=1  LatchInput=off
  Enable : EnablePort
  AB_LEVEL : Constant  Value=ab_level
  ALPFA_BETA_SUM : Fcn  Expr=sqrt(u[1]^2+u[2]^2)
  ALPFA_BETA_SUM1 : Fcn  Expr=abs(u[3]) * 3
  C : Constant  Value=filt_tc
  C1 : Constant  Value=1/(fn)
  CLARK : Subsystem  AncestorBlock=lib_mesures/CLARK
  Gain : Gain  Gain=ab_gain  SaturateOnIntegerOverflow=on
  "Gain  " : Gain  Gain=z_gain  SaturateOnIntegerOverflow=on
  Ground : Ground
  LP T= 0.03 : powerlib_extras/Discrete  Control Blocks/Discrete 1st-Order Discrete Filter  FilterType=Lowpass  Tc=0.03  Ts=Ts  Initialize=off  Vac_Init=[0.8 -25 60]*0  Vdc_Init=filt_ic  PlotResponse=off  param1=[1 500 0.1]
  Max: 1 pu Min = 0 : Saturate  UpperLimit=1.0  LowerLimit=0
  MinMax1 : MinMax  Function=max  SaturateOnIntegerOverflow=on  InputSameDT=on
  MinMax2 : MinMax  Function=max  SaturateOnIntegerOverflow=on  InputSameDT=on
  MinMax3 : MinMax  Function=max  Inputs=2  SaturateOnIntegerOverflow=on  InputSameDT=on
  MinMax4 : MinMax  Function=max  Inputs=2  SaturateOnIntegerOverflow=on  InputSameDT=on
  PB_R : Subsystem  mask(Low Pass Filter With Reset (discrete: Zoh method, Forward Euler)){ic=1, dt=Ts}
      mask prompts: ic "Initial condition:"; dt "Sample time (s)"
      mask help:
      | The output will be reset to the input value (Time constant = 0)  during the input (2) is True. The Time constant (T) is defined by
      | input (3).
      mask Display:
      | plot(0,0,100,100,[90,80,70,60,50,40,29,20,10],[60,55,52,55,60,65,67,65,60],[89,80,71,60,50,40,30,20,10],[40,35,32,35,40,45,47,45,40],[56,44],[70,50]);
      | disp('\n\nD')
  Relational Operator : RelationalOperator  Operator=>
  Relational Operator1 : RelationalOperator  Operator=>
  Sum : Sum  Inputs=+-  SaturateOnIntegerOverflow=on
  Switch : Switch  Threshold=0.5  SaturateOnIntegerOverflow=on
  Switch1 : Switch  Threshold=0.5  SaturateOnIntegerOverflow=on
  Switch2 : Switch  Threshold=0.5  SaturateOnIntegerOverflow=on
  T_PERIODE : Subsystem  AncestorBlock=powerlib_extras/Discrete Measurements/FFT/Averager1  mask(Shift Register with discrete state space block){Navg=fix(T_periode/Ts), x0=0, Ts=Ts}
      mask prompts: Navg "Number of Samples inl. in(k)"; x0 "Inititial Condition"; Ts "Sample Time (-1 for inherited)"
      mask help: This block is a shift register storing values [u(k) u(k-1) ... u(k-(Navg-1))]' . This vector can be used for a FFT analysis.
      mask init:
      | %Discrete State Space model of averager
      | %one scalar input
      | %Navg sized output [in(k) in(k-1) .... in(k-(Navg-1))]
      | Q=eye(Navg-1);
      | A=[Q(:,2:length(Q))  Q(:,1)] ;
      | A(1,Navg-1)=0;
      | B=[1 ; zeros(Navg-2,1)];
      | C=eye(Navg) ;
      | C=C(:,2:length(C));
      | D=[1 ; zeros(Navg-1,1)];
      mask Help: This block is a shift register storing values [u(k) u(k-1) ... u(k-(Navg-1))]' . This vector can be used for a FFT analysis.
      mask Display: disp('Shift\nRegister')
  "T_PERIODE " : Subsystem  AncestorBlock=powerlib_extras/Discrete Measurements/FFT/Averager1  mask(Shift Register with discrete state space block){Navg=fix(T_periode/Ts), x0=0, Ts=Ts}
      mask prompts: Navg "Number of Samples inl. in(k)"; x0 "Inititial Condition"; Ts "Sample Time (-1 for inherited)"
      mask help: This block is a shift register storing values [u(k) u(k-1) ... u(k-(Navg-1))]' . This vector can be used for a FFT analysis.
      mask init: same as power_hvdc12pulse/Inverter Control and Protection/Inverter Protections/Commutation Failure Prevention Control (CFPREV)/Enabled Subsystem/T_PERIODE
      mask Help: This block is a shift register storing values [u(k) u(k-1) ... u(k-(Navg-1))]' . This vector can be used for a FFT analysis.
      mask Display: disp('Shift\nRegister')
  T_ss : Step  Time=T_ss  Before=1  After=0  SampleTime=0
  ZERO : Constant  Value=0
  ZERO1 : Constant  Value=0
  Z_LEVEL : Constant  Value=z_level
  AMIN_CFPREV (deg) : Outport
  wires:
  MinMax4/1 -> AMIN_CFPREV (deg)/1
  LP T= 0.03/1 -> MinMax4/1
  MinMax3/1 -> LP T= 0.03/1, MinMax4/2
  ALPFA_BETA_SUM/1 -> Sum/2, PB_R/1("In ")
  Sum/1 -> "T_PERIODE "/1(u), Relational Operator/1
  AB_LEVEL/1 -> Relational Operator/2
  Relational Operator/1 -> Switch/2  "AB_DET"
  "T_PERIODE "/1("[u;x]") -> MinMax1/1
  MinMax1/1 -> Gain/1
  Gain/1 -> Switch/1  "AB_AMIN"
  ZERO/1 -> Switch/3
  ALPFA_BETA_SUM1/1 -> Relational Operator1/1, T_PERIODE/1(u)  "Z_DIFF"
  Z_LEVEL/1 -> Relational Operator1/2
  T_PERIODE/1("[u;x]") -> MinMax2/1
  MinMax2/1 -> Max: 1 pu Min = 0/1
  Max: 1 pu Min = 0/1 -> "Gain  "/1
  Relational Operator1/1 -> Switch1/2  "Z_DET"
  "Gain  "/1 -> Switch1/1  "Z_AMIN"
  ZERO1/1 -> Switch1/3
  Switch/1 -> MinMax3/1  "AB MIN"
  Switch1/1 -> MinMax3/2  "Z MIN"
  CLARK/1(ab0) -> ALPFA_BETA_SUM/1, ALPFA_BETA_SUM1/1
  Uabc (pu)/1 -> CLARK/1(abc)
  PB_R/1(Out) -> Sum/1
  Switch2/1 -> PB_R/3(T)
  C/1 -> Switch2/3
  T_ss/1 -> Switch2/2
  C1/1 -> Switch2/1
  Ground/1 -> PB_R/2(Reset)

== system power_hvdc12pulse/Inverter Control and Protection/Inverter Protections/Low AC Voltage Detection (LACVD)/Enabled Subsystem ==
  note: Silvano Casoria
      | Power System Laboratory, IREQ
      | Hydro-Quebec
  note: Low AC Voltage Detection
  Uac (pu) : Inport  Port=1  LatchInput=off
  Enable : EnablePort
  "Off Delay " : powerlib_extras/Discrete  Control Blocks/Discrete On//Off Delay  type_delay=Off delay  delay=0.009  ic=0  Ts=dt
  On Delay : powerlib_extras/Discrete  Control Blocks/Discrete On//Off Delay  type_delay=On delay  delay=0.014  ic=0  Ts=dt
  "On Delay " : powerlib_extras/Discrete  Control Blocks/Discrete On//Off Delay  type_delay=On delay  delay=0.001  ic=0  Ts=dt
  REF 1 (pu) : Constant  Value=Ref_1
  Relational Operator1 : RelationalOperator  Operator=<=  InputSameDT=on
  Low_AC_Voltage : Outport
  wires:
  Relational Operator1/1 -> "On Delay "/1
  "On Delay "/1 -> "Off Delay "/1
  "Off Delay "/1 -> On Delay/1
  REF 1 (pu)/1 -> Relational Operator1/2
  On Delay/1 -> Low_AC_Voltage/1
  Uac (pu)/1 -> Relational Operator1/1

== system power_hvdc12pulse/Rectifier Control and Protection/12-pulse Firing Control1/Discrete Synchronized 12-Pulse Generator/12 Flip-Flops ==
  S : Inport  Port=1  LatchInput=off
  R : Inport  Port=2  LatchInput=off
  6 Flip-Flop : Subsystem
  6 Flip-Flop1 : Subsystem
  Demux : Demux  Outputs=2
  Demux1 : Demux  Outputs=2
  Mux : Mux  Inputs=2
  Q : Outport
  wires:
  S/1 -> Demux/1
  Demux/1 -> 6 Flip-Flop/1(S)
  Demux/2 -> 6 Flip-Flop1/1(S)
  R/1 -> Demux1/1
  Demux1/2 -> 6 Flip-Flop1/2(R)
  Demux1/1 -> 6 Flip-Flop/2(R)
  6 Flip-Flop/1(Q) -> Mux/1
  Mux/1 -> Q/1
  6 Flip-Flop1/1(Q) -> Mux/2

== system power_hvdc12pulse/Rectifier Control and Protection/Rectifier Protections/DC Fault Protection (DCPROT)/Enabled Subsystem ==
  note: Silvano Casoria
      | Power System Laboratory, IREQ
      | Hydro-Quebec
  note: DC Fault Protection (only in Rectifier)
  VdL (pu) : Inport  Port=1  LatchInput=off
  Deblocked : Inport  Port=2  DataType=boolean  LatchInput=off
  Lock : Inport  Port=3  LatchInput=off
  Enable : EnablePort
  Data Type Conversion : DataTypeConversion  OutDataTypeMode=boolean  SaturateOnIntegerOverflow=on  RndMeth=Zero
  Discrete Off Delay : powerlib_extras/Discrete  Control Blocks/Discrete On//Off Delay  type_delay=Off delay  delay=0.160  ic=0  Ts=dt
  "Discrete On Delay  " : powerlib_extras/Discrete  Control Blocks/Discrete On//Off Delay  type_delay=On delay  delay=0.2  ic=0  Ts=dt
  Logical Operator2 : Logic  Inputs=3
  Logical Operator3 : Logic  Operator=NOT
  Logical Operator6 : Logic
  "Monostable: T2 " : powerlib_extras/Discrete  Control Blocks/Discrete Monostable  EdgeDetect=Rising  t_mono=T2  ic=0  Ts=dt
  "Off Delay " : powerlib_extras/Discrete  Control Blocks/Discrete On//Off Delay  type_delay=Off delay  delay=0.01  ic=0  Ts=dt
  On Delay: T1 : powerlib_extras/Discrete  Control Blocks/Discrete On//Off Delay  type_delay=On delay  delay=T1  ic=0  Ts=dt
  Ref1 (pu) : Relay  OnSwitchValue=-Ref1  OffSwitchValue=-(Ref1 + 0.1)
  minus : Gain  Gain=-1  SaturateOnIntegerOverflow=on
  voltage sign (pole +) : Gain  Gain=sign  SaturateOnIntegerOverflow=on
  Forced_alpha : Outport
  wires:
  minus/1 -> Ref1 (pu)/1
  Data Type Conversion/1 -> Logical Operator6/1
  "Discrete On Delay  "/1 -> Logical Operator6/2
  Logical Operator6/1 -> "Off Delay "/1
  Ref1 (pu)/1 -> Data Type Conversion/1
  Deblocked/1 -> Logical Operator2/3, "Discrete On Delay  "/1
  VdL (pu)/1 -> voltage sign (pole +)/1  "VdL"
  voltage sign (pole +)/1 -> minus/1
  Lock/1 -> Discrete Off Delay/1
  "Off Delay "/1 -> Logical Operator2/1
  Discrete Off Delay/1 -> Logical Operator3/1
  Logical Operator3/1 -> Logical Operator2/2
  Logical Operator2/1 -> On Delay: T1/1
  On Delay: T1/1 -> "Monostable: T2 "/1
  "Monostable: T2 "/1 -> Forced_alpha/1

== system power_hvdc12pulse/Rectifier Control and Protection/Rectifier Protections/Low AC Voltage Detection (LACVD)/Enabled Subsystem ==
  note: Silvano Casoria
      | Power System Laboratory, IREQ
      | Hydro-Quebec
  note: Low AC Voltage Detection
  Uac (pu) : Inport  Port=1  LatchInput=off
  Enable : EnablePort
  "Off Delay " : powerlib_extras/Discrete  Control Blocks/Discrete On//Off Delay  type_delay=Off delay  delay=0.009  ic=0  Ts=dt
  On Delay : powerlib_extras/Discrete  Control Blocks/Discrete On//Off Delay  type_delay=On delay  delay=0.014  ic=0  Ts=dt
  "On Delay " : powerlib_extras/Discrete  Control Blocks/Discrete On//Off Delay  type_delay=On delay  delay=0.001  ic=0  Ts=dt
  REF 1 (pu) : Constant  Value=Ref_1
  Relational Operator1 : RelationalOperator  Operator=<=  InputSameDT=on
  Low_AC_Voltage : Outport
  wires:
  Relational Operator1/1 -> "On Delay "/1
  "On Delay "/1 -> "Off Delay "/1
  "Off Delay "/1 -> On Delay/1
  REF 1 (pu)/1 -> Relational Operator1/2
  On Delay/1 -> Low_AC_Voltage/1
  Uac (pu)/1 -> Relational Operator1/1

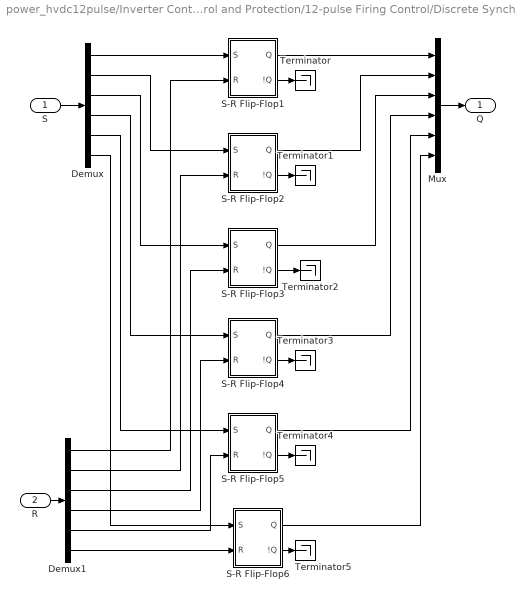
== system power_hvdc12pulse/Inverter Control and Protection/12-pulse Firing Control/Discrete Synchronized 12-Pulse Generator/12 Flip-Flops/6 Flip-Flop ==
  S : Inport  Port=1  LatchInput=off
  R : Inport  Port=2  LatchInput=off
  Demux : Demux  Outputs=6
  Demux1 : Demux  Outputs=6
  Mux : Mux  Inputs=6
  S-R Flip-Flop1 : Subsystem  mask(SRFlipFlop){initial_condition=0, Ts=Ts}
      mask prompts: initial_condition "Initial condition:"; Ts "Sample time:"
      mask help: S-R Flip Flop Block
  S-R Flip-Flop2 : Subsystem  mask(SRFlipFlop){initial_condition=0, Ts=Ts}
      mask prompts: initial_condition "Initial condition:"; Ts "Sample time:"
      mask help: S-R Flip Flop Block
  S-R Flip-Flop3 : Subsystem  mask(SRFlipFlop){initial_condition=0, Ts=Ts}
      mask prompts: initial_condition "Initial condition:"; Ts "Sample time:"
      mask help: S-R Flip Flop Block
  S-R Flip-Flop4 : Subsystem  mask(SRFlipFlop){initial_condition=0, Ts=Ts}
      mask prompts: initial_condition "Initial condition:"; Ts "Sample time:"
      mask help: S-R Flip Flop Block
  S-R Flip-Flop5 : Subsystem  mask(SRFlipFlop){initial_condition=0, Ts=Ts}
      mask prompts: initial_condition "Initial condition:"; Ts "Sample time:"
      mask help: S-R Flip Flop Block
  S-R Flip-Flop6 : Subsystem  mask(SRFlipFlop){initial_condition=0, Ts=Ts}
      mask prompts: initial_condition "Initial condition:"; Ts "Sample time:"
      mask help: S-R Flip Flop Block
  Terminator{,1..5} (6 alike) : Terminator
  Q : Outport
  wires:
  S-R Flip-Flop6/2(!Q) -> Terminator5/1
  S-R Flip-Flop5/2(!Q) -> Terminator4/1
  S-R Flip-Flop4/2(!Q) -> Terminator3/1
  S-R Flip-Flop3/2(!Q) -> Terminator2/1
  S-R Flip-Flop2/2(!Q) -> Terminator1/1
  S-R Flip-Flop1/1(Q) -> Mux/1
  S-R Flip-Flop2/1(Q) -> Mux/2
  S-R Flip-Flop3/1(Q) -> Mux/3
  S-R Flip-Flop4/1(Q) -> Mux/4
  S-R Flip-Flop5/1(Q) -> Mux/5
  Mux/1 -> Q/1
  S-R Flip-Flop6/1(Q) -> Mux/6
  S-R Flip-Flop1/2(!Q) -> Terminator/1
  Demux/1 -> S-R Flip-Flop1/1(S)
  Demux/2 -> S-R Flip-Flop2/1(S)
  Demux/3 -> S-R Flip-Flop3/1(S)
  Demux/4 -> S-R Flip-Flop4/1(S)
  S/1 -> Demux/1
  Demux/6 -> S-R Flip-Flop6/1(S)
  Demux/5 -> S-R Flip-Flop5/1(S)
  R/1 -> Demux1/1
  Demux1/1 -> S-R Flip-Flop1/2(R)
  Demux1/2 -> S-R Flip-Flop2/2(R)
  Demux1/3 -> S-R Flip-Flop3/2(R)
  Demux1/4 -> S-R Flip-Flop4/2(R)
  Demux1/5 -> S-R Flip-Flop5/2(R)
  Demux1/6 -> S-R Flip-Flop6/2(R)
